simulink model "crane_model_v02_sim_improved"  (R2021a)
settings: Solver=ode23t  StartTime=0.0  StopTime=120.0  RelTol=1e-3
model workspace (MAT data in the model file):
  I_xx_0 = Simulink.Parameter
  I_xx_0.Value = 300
  I_xx_0.DataType = 'auto'
  I_xx_0.DocUnits = 'kg*m*m'
  I_xx_0.Dimensions = [1 1]
  I_xx_1 = Simulink.Parameter
  I_xx_1.Value = 336.25
  I_xx_1.DataType = 'auto'
  I_xx_1.DocUnits = 'kg*m*m'
  I_xx_1.Dimensions = [1 1]
  I_xx_2 = Simulink.Parameter
  I_xx_2.Value = 313.83
  I_xx_2.DataType = 'auto'
  I_xx_2.DocUnits = 'kg*m*m'
  I_xx_2.Dimensions = [1 1]
  I_xx_b = Simulink.Parameter
  I_xx_b.Value = 12.917
  I_xx_b.DataType = 'auto'
  I_xx_b.DocUnits = 'kg*m*m'
  I_xx_b.Dimensions = [1 1]
  I_xx_b1 = Simulink.Parameter
  I_xx_b1.Value = 10.905
  I_xx_b1.DataType = 'auto'
  I_xx_b1.Dimensions = [1 1]
  I_xx_b2 = Simulink.Parameter
  I_xx_b2.Value = 7.1406
  I_xx_b2.DataType = 'auto'
  I_xx_b2.Dimensions = [1 1]
  I_xx_c1 = Simulink.Parameter
  I_xx_c1.Value = 4.2383
  I_xx_c1.DataType = 'auto'
  I_xx_c1.Dimensions = [1 1]
  I_xx_c2 = Simulink.Parameter
  I_xx_c2.Value = 2.474
  I_xx_c2.DataType = 'auto'
  I_xx_c2.Dimensions = [1 1]
  I_yy_0 = Simulink.Parameter
  I_yy_0.Value = 300
  I_yy_0.DataType = 'auto'
  I_yy_0.DocUnits = 'kg*m*m'
  I_yy_0.Dimensions = [1 1]
  I_yy_1 = Simulink.Parameter
  I_yy_1.Value = 336.25
  I_yy_1.DataType = 'auto'
  I_yy_1.DocUnits = 'kg*m*m'
  I_yy_1.Dimensions = [1 1]
  I_yy_2 = Simulink.Parameter
  I_yy_2.Value = 313.83
  I_yy_2.DataType = 'auto'
  I_yy_2.DocUnits = 'kg*m*m'
  I_yy_2.Dimensions = [1 1]
  I_yy_b = Simulink.Parameter
  I_yy_b.Value = 12.917
  I_yy_b.DataType = 'auto'
  I_yy_b.DocUnits = 'kg*m*m'
  I_yy_b.Dimensions = [1 1]
  I_yy_b1 = Simulink.Parameter
  I_yy_b1.Value = 10.905
  I_yy_b1.DataType = 'auto'
  I_yy_b1.Dimensions = [1 1]
  I_yy_b2 = Simulink.Parameter
  I_yy_b2.Value = 7.1406
  I_yy_b2.DataType = 'auto'
  I_yy_b2.Dimensions = [1 1]
  I_yy_c1 = Simulink.Parameter
  I_yy_c1.Value = 4.2383
  I_yy_c1.DataType = 'auto'
  I_yy_c1.Dimensions = [1 1]
  I_yy_c2 = Simulink.Parameter
  I_yy_c2.Value = 2.474
  I_yy_c2.DataType = 'auto'
  I_yy_c2.Dimensions = [1 1]
  I_zz_0 = Simulink.Parameter
  I_zz_0.Value = 12
  I_zz_0.DataType = 'auto'
  I_zz_0.DocUnits = 'kg*m*m'
  I_zz_0.Dimensions = [1 1]
  I_zz_1 = Simulink.Parameter
  I_zz_1.Value = 11.25
  I_zz_1.DataType = 'auto'
  I_zz_1.DocUnits = 'kg*m*m'
  I_zz_1.Dimensions = [1 1]
  I_zz_2 = Simulink.Parameter
  I_zz_2.Value = 10.5
  I_zz_2.DataType = 'auto'
  I_zz_2.DocUnits = 'kg*m*m'
  I_zz_2.Dimensions = [1 1]
  I_zz_b = Simulink.Parameter
  I_zz_b.Value = 11.25
  I_zz_b.DataType = 'auto'
  I_zz_b.DocUnits = 'kg*m*m'
  I_zz_b.Dimensions = [1 1]
  I_zz_b1 = Simulink.Parameter
  I_zz_b1.Value = 0.16276
  I_zz_b1.DataType = 'auto'
  I_zz_b1.Dimensions = [1 1]
  I_zz_b2 = Simulink.Parameter
  I_zz_b2.Value = 0.13021
  I_zz_b2.DataType = 'auto'
  I_zz_b2.Dimensions = [1 1]
  I_zz_c1 = Simulink.Parameter
  I_zz_c1.Value = 0.16276
  I_zz_c1.DataType = 'auto'
  I_zz_c1.Dimensions = [1 1]
  I_zz_c2 = Simulink.Parameter
  I_zz_c2.Value = 0.13021
  I_zz_c2.DataType = 'auto'
  I_zz_c2.Dimensions = [1 1]
  J_a = Simulink.Parameter
  J_a.Value = 3.125
  J_a.DataType = 'auto'
  J_a.DocUnits = 'kg*m*m'
  J_a.Dimensions = [1 1]
  Sig = Simulink.Signal
  Sig.DataType = 'auto'
  Sig.Dimensions = -1
  Sig.DimensionsMode = 'auto'
  Sig.Complexity = 'auto'
  Sig.SampleTime = -1
  Sig.SamplingMode = 'auto'
  Sig1 = Simulink.Signal
  Sig1.DataType = 'auto'
  Sig1.Dimensions = -1
  Sig1.DimensionsMode = 'auto'
  Sig1.Complexity = 'auto'
  Sig1.SampleTime = -1
  Sig1.SamplingMode = 'auto'
  a1_l = Simulink.Parameter
  a1_l.Value = Simulink.data.Expression
  a1_l.Value.ExpressionString = "sqrt((l_0-h_base-l_b4y)^2+(l_b4x-l_b1x)^2)"
  a1_l.DataType = 'auto'
  a1_l.Dimensions = -1
  a1_t = Simulink.Parameter
  a1_t.Value = Simulink.data.Expression
  a1_t.Value.ExpressionString = "atan((l_0-h_base-l_b4y)/(l_b4x-l_b1x))"
  a1_t.DataType = 'auto'
  a1_t.Dimensions = -1
  a2_l = Simulink.Parameter
  a2_l.Value = Simulink.data.Expression
  a2_l.Value.ExpressionString = "sqrt((l_c1x-l_c3y)^2+(l_c3x-l_c1y)^2)"
  a2_l.DataType = 'auto'
  a2_l.Dimensions = -1
  a2_t = Simulink.Parameter
  a2_t.Value = Simulink.data.Expression
  a2_t.Value.ExpressionString = "atan((l_c1x-l_c3y)/(l_c3x-l_c1y))"
  a2_t.DataType = 'auto'
  a2_t.Dimensions = -1
  arm_d = Simulink.Parameter
  arm_d.Value = 0.3
  arm_d.DataType = 'auto'
  arm_d.DocUnits = 'm'
  arm_d.Dimensions = [1 1]
  arm_w = Simulink.Parameter
  arm_w.Value = 0.3
  arm_w.DataType = 'auto'
  arm_w.DocUnits = 'm'
  arm_w.Dimensions = [1 1]
  b_1 = Simulink.Parameter
  b_1.Value = Simulink.data.Expression
  b_1.Value.ExpressionString = "sqrt(l_b1x^2+(l_0-l_b1x)^2)"
  b_1.DataType = 'auto'
  b_1.DocUnits = 'm'
  b_1.Dimensions = -1
  b_2 = Simulink.Parameter
  b_2.Value = Simulink.data.Expression
  b_2.Value.ExpressionString = "sqrt(l_c3x^2+l_c3y^2)"
  b_2.DataType = 'auto'
  b_2.DocUnits = 'm'
  b_2.Dimensions = -1
  h_base = Simulink.Parameter
  h_base.Value = 0.2
  h_base.DataType = 'auto'
  h_base.DocUnits = 'm'
  h_base.Dimensions = [1 1]
  l_0 = Simulink.Parameter
  l_0.Value = 2.1
  l_0.DataType = 'auto'
  l_0.DocUnits = 'm'
  l_0.Dimensions = [1 1]
  l_1 = Simulink.Parameter
  l_1.Value = 2.3
  l_1.DataType = 'auto'
  l_1.DocUnits = 'm'
  l_1.Dimensions = [1 1]
  l_2 = Simulink.Parameter
  l_2.Value = 2.1
  l_2.DataType = 'auto'
  l_2.DocUnits = 'm'
  l_2.Dimensions = [1 1]
  l_a1_rod = Simulink.Parameter
  l_a1_rod.Value = Simulink.data.Expression
  l_a1_rod.Value.ExpressionString = "a1_l-l_b2"
  l_a1_rod.DataType = 'auto'
  l_a1_rod.DocUnits = 'm'
  l_a1_rod.Dimensions = -1
  l_a2_rod = Simulink.Parameter
  l_a2_rod.Value = Simulink.data.Expression
  l_a2_rod.Value.ExpressionString = "a2_l-l_c2"
  l_a2_rod.DataType = 'auto'
  l_a2_rod.DocUnits = 'm'
  l_a2_rod.Dimensions = -1
  l_b1x = Simulink.Parameter
  l_b1x.Value = 0.3
  l_b1x.DataType = 'auto'
  l_b1x.DocUnits = 'm'
  l_b1x.Dimensions = [1 1]
  l_b1z = Simulink.Parameter
  l_b1z.Value = 0.2
  l_b1z.DataType = 'auto'
  l_b1z.DocUnits = 'm'
  l_b1z.Dimensions = [1 1]
  l_b2 = Simulink.Parameter
  l_b2.Value = 1
  l_b2.DataType = 'auto'
  l_b2.DocUnits = 'm'
  l_b2.Dimensions = [1 1]
  l_b4x = Simulink.Parameter
  l_b4x.Value = 0.5
  l_b4x.DataType = 'auto'
  l_b4x.DocUnits = 'm'
  l_b4x.Dimensions = [1 1]
  l_b4y = Simulink.Parameter
  l_b4y.Value = 0.15
  l_b4y.DataType = 'auto'
  l_b4y.DocUnits = 'm'
  l_b4y.Dimensions = [1 1]
  l_c1x = Simulink.Parameter
  l_c1x.Value = 1.1
  l_c1x.DataType = 'auto'
  l_c1x.DocUnits = 'm'
  l_c1x.Dimensions = [1 1]
  l_c1y = Simulink.Parameter
  l_c1y.Value = 0.15
  l_c1y.DataType = 'auto'
  l_c1y.DocUnits = 'm'
  l_c1y.Dimensions = [1 1]
  l_c2 = Simulink.Parameter
  l_c2.Value = 0.6
  l_c2.DataType = 'auto'
  l_c2.DocUnits = 'm'
  l_c2.Dimensions = [1 1]
  l_c3x = Simulink.Parameter
  l_c3x.Value = 0.65
  l_c3x.DataType = 'auto'
  l_c3x.DocUnits = 'm'
  l_c3x.Dimensions = [1 1]
  l_c3y = Simulink.Parameter
  l_c3y.Value = 0.15
  l_c3y.DataType = 'auto'
  l_c3y.DocUnits = 'm'
  l_c3y.Dimensions = [1 1]
  l_set = 0.5
  m_0 = Simulink.Parameter
  m_0.Value = 800
  m_0.DataType = 'auto'
  m_0.DocUnits = 'kg'
  m_0.Dimensions = [1 1]
  m_1 = Simulink.Parameter
  m_1.Value = 750
  m_1.DataType = 'auto'
  m_1.DocUnits = 'kg'
  m_1.Dimensions = [1 1]
  m_2 = Simulink.Parameter
  m_2.Value = 700
  m_2.DataType = 'auto'
  m_2.DocUnits = 'kg'
  m_2.Dimensions = [1 1]
  m_b1 = Simulink.Parameter
  m_b1.Value = 125
  m_b1.DataType = 'auto'
  m_b1.DocUnits = 'kg'
  m_b1.Dimensions = [1 1]
  m_b2 = Simulink.Parameter
  m_b2.Value = 100
  m_b2.DataType = 'auto'
  m_b2.DocUnits = 'kg'
  m_b2.Dimensions = [1 1]
  m_base = Simulink.Parameter
  m_base.Value = 500
  m_base.DataType = 'auto'
  m_base.DocUnits = 'kg'
  m_base.Dimensions = [1 1]
  m_c1 = Simulink.Parameter
  m_c1.Value = 125
  m_c1.DataType = 'auto'
  m_c1.DocUnits = 'kg'
  m_c1.Dimensions = [1 1]
  m_c2 = Simulink.Parameter
  m_c2.Value = 100
  m_c2.DataType = 'auto'
  m_c2.DocUnits = 'kg'
  m_c2.Dimensions = [1 1]
  m_p = Simulink.Parameter
  m_p.Value = 2000
  m_p.DataType = 'auto'
  m_p.DocUnits = 'kg'
  m_p.Dimensions = [1 1]
  r_base = Simulink.Parameter
  r_base.Value = 0.3
  r_base.DataType = 'auto'
  r_base.DocUnits = 'm'
  r_base.Dimensions = [1 1]
  r_cyl = Simulink.Parameter
  r_cyl.Value = 0.125
  r_cyl.DataType = 'auto'
  r_cyl.DocUnits = 'm'
  r_cyl.Dimensions = [1 1]
  r_cyl_0 = Simulink.Parameter
  r_cyl_0.Value = 0.1
  r_cyl_0.DataType = 'auto'
  r_cyl_0.Dimensions = [1 1]
  x_set = 3.7
  y_set = 0.3
  z_set = 2.2
undefined symbols (not defined in the file): sigbuilder_block, X, Y, Z
libraries: sm_lib x103, nesl_utility x23, pid_lib x7, fuzblock x1
(part 1 of 5)
settings Model: OrderedModelArguments=off  Creator=jjmoey  LastModifiedBy=jjmoey

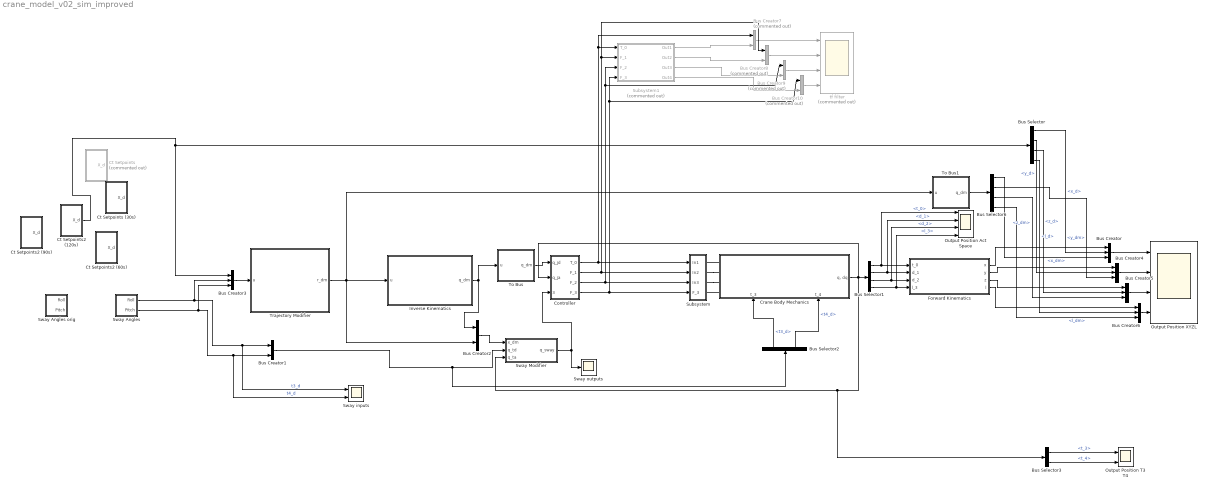
== system crane_model_v02_sim_improved ==
  Bus Creator{,3..6} (5 alike) : BusCreator  Inputs=3
  Bus Creator1 : BusCreator  Inputs=2
  Bus Creator{7..10} (4 alike) : BusCreator  Commented=on  Inputs=2
  Bus Creator2 : BusCreator  Inputs=2
  Bus Selector : BusSelector  OutputSignals=x_d,y_d,z_d,l_d
  Bus Selector1 : BusSelector  OutputSignals=t_0,d_1,d_2,l_3
  Bus Selector2 : BusSelector  OutputSignals=t3_d,t4_d
  Bus Selector3 : BusSelector  OutputSignals=t_3,t_4
  Bus Selector6 : BusSelector  OutputSignals=x_dm,y_dm,z_dm,l_dm
  Controller : Subsystem
  Crane Body Mechanics : Subsystem
      settings: PortSchema="{\"entries\":[{\"content\":{\"sides\":[{\"content\":{\"connectorIds\":[\"LConn1\",\"LConn2\",\"LConn3\",\"LConn4\"]},\"type\":\"ConnectorPlacement.EquallySpacedRectSide\",\"uuid\":\"3c12a75b-c014-4331-843e-93cd976182ad\"},{\"content\":{\"connectorIds\":[\"Out1\"],\"side\":\"RIGHT\"},\"type\":\"ConnectorPlacement.EquallySpacedRectSide\",\"uuid\":\"f6a8e3a7-cb13-4e9f-a0f7-1b13ae567996\"},{\"content\":{\"connectorIds\":[],\"side\":\"TOP\"},\"type\":\"ConnectorPlacement.EquallySpacedRectSide\",\"uuid\":\"21d4657c-d1b0-4888-a00c-4d42a03474ee\"},{\"content\":{\"connectorIds\":[\"In1\",\"In2\"],\"side\":\"BOTTOM\"},\"type\":\"ConnectorPlacement.EquallySpacedRectSide\",\"uuid\":\"dc246dea-fc9c-4a87-b817-efe1b28a592a\"}]},\"type\":\"ConnectorPlacement.EquallySpacedConnector\",\"uuid\":\"e18ee79d-7142-4697-ae33-8ae8c5e54180\"}],\"packageUris\":[\"http://schema.mathworks.com/mf0/Connector/R2020b\"],\"version\":\"1.0\"}"
  Ct Setpoints : Subsystem  Commented=on
  Ct Setpoints (30s) : Subsystem
  Ct Setpoints2 (120s) : Subsystem
  Ct Setpoints2 (60s) : Subsystem
  Ct Setpoints2 (90s) : Subsystem
  Forward Kinematics : MATLAB Function  TreatAsAtomicUnit=on
  Inverse Kinematics : MATLAB Function  TreatAsAtomicUnit=on
  Output Position Act Space : Scope  NumInputPorts=4
  Output Position T3 T4 : Scope  NumInputPorts=2
  Output Position XYZL : Scope  NumInputPorts=4
  Subsystem : Subsystem
  Subsystem1 : Subsystem  Commented=on
  Sway Angles : Subsystem
  Sway Angles orig : Subsystem
  Sway Modifier : Subsystem
  Sway inputs : Scope  NumInputPorts=2
  Sway outputs : Scope
  To Bus : Subsystem
  To Bus1 : Subsystem
  Trajectory Modifier : MATLAB Function  TreatAsAtomicUnit=on
  tf filter : Scope  Commented=on  NumInputPorts=4
  wires:
  Sway Angles/1(Roll) -> Bus Creator3/2, Sway inputs/1, Bus Creator1/1  "t3_d"
  Sway Angles/2(Pitch) -> Bus Creator3/3, Sway inputs/2, Bus Creator1/2  "t4_d"
  Ct Setpoints2 (120s)/1(X_d) -> Bus Creator3/1, Bus Selector/1
  Inverse Kinematics/1(q_dm) -> To Bus/1(u), Bus Creator2/1
  Crane Body Mechanics/1("q, dq") -> Bus Selector3/1, Sway Modifier/3(q_ta), Controller/2(q_ja), Bus Selector1/1
  Bus Selector1/1 -> Output Position Act Space/1, Forward Kinematics/1(t_0)  "<t_0>"
  Bus Selector1/2 -> Output Position Act Space/2, Forward Kinematics/2(d_1)  "<d_1>"
  Bus Selector1/3 -> Output Position Act Space/3, Forward Kinematics/3(d_2)  "<d_2>"
  Bus Selector1/4 -> Output Position Act Space/4, Forward Kinematics/4(l_3)  "<l_3>"
  Bus Creator2/1 -> Sway Modifier/1(x_dm)
  Sway Modifier/1(q_sway) -> Sway outputs/1, Controller/3(q_sway)
  Bus Creator3/1 -> Trajectory Modifier/1(u)
  To Bus/1(q_dm) -> Controller/1(q_jd)
  Trajectory Modifier/1(r_dm) -> Bus Creator2/2, To Bus1/1(u), Inverse Kinematics/1(u)
  Forward Kinematics/1(x) -> Bus Creator/1
  Bus Selector/1 -> Bus Creator/2  "<x_d>"
  Bus Selector6/1 -> Bus Creator/3  "<x_dm>"
  To Bus1/1(q_dm) -> Bus Selector6/1
  Bus Creator/1 -> Output Position XYZL/1
  Bus Creator6/1 -> Output Position XYZL/4
  Bus Creator5/1 -> Output Position XYZL/3
  Bus Creator4/1 -> Output Position XYZL/2
  Bus Selector/2 -> Bus Creator4/2  "<y_d>"
  Bus Selector6/2 -> Bus Creator4/3  "<y_dm>"
  Forward Kinematics/2(y) -> Bus Creator4/1
  Forward Kinematics/3(z) -> Bus Creator5/1
  Bus Selector6/3 -> Bus Creator5/3  "<z_dm>"
  Bus Selector/3 -> Bus Creator5/2  "<z_d>"
  Forward Kinematics/4(l) -> Bus Creator6/1
  Bus Selector/4 -> Bus Creator6/2  "<l_d>"
  Bus Selector6/4 -> Bus Creator6/3  "<l_dm>"
  Bus Creator1/1 -> Bus Selector2/1, Sway Modifier/2(q_td)
  Bus Selector2/1 -> Crane Body Mechanics/1(t_3)  "<t3_d>"
  Bus Selector2/2 -> Crane Body Mechanics/2(t_4)  "<t4_d>"
  Bus Selector3/1 -> Output Position T3 T4/1  "<t_3>"
  Bus Selector3/2 -> Output Position T3 T4/2  "<t_4>"
  Bus Creator10/1 -> tf filter/4
  Bus Creator9/1 -> tf filter/3
  Bus Creator8/1 -> tf filter/2
  Bus Creator7/1 -> tf filter/1
  Controller/1(T_0) -> Bus Creator7/1, Subsystem1/1(T_0), Subsystem/1(In1)
  Controller/2(F_1) -> Bus Creator8/1, Subsystem1/2(F_1), Subsystem/2(In2)
  Controller/3(F_2) -> Subsystem1/3(F_2), Bus Creator9/1, Subsystem/3(In3)
  Controller/4(F_3) -> Subsystem1/4(F_3), Bus Creator10/1, Subsystem/4(F_3)
  Subsystem1/1(Out1) -> Bus Creator7/2
  Subsystem1/2(Out2) -> Bus Creator8/2
  Subsystem1/3(Out3) -> Bus Creator9/2
  Subsystem1/4(Out4) -> Bus Creator10/2
  connections:
  Crane Body Mechanics/LConn1 -- Subsystem/RConn1
  Subsystem/RConn3 -- Crane Body Mechanics/LConn3
  Subsystem/RConn2 -- Crane Body Mechanics/LConn2
  Crane Body Mechanics/LConn4 -- Subsystem/RConn4

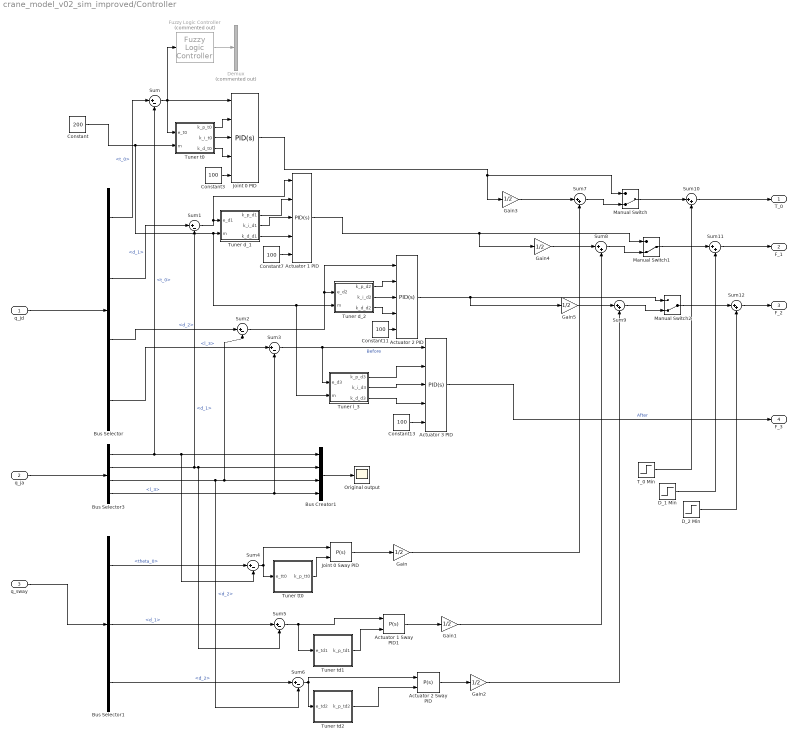
== system crane_model_v02_sim_improved/Controller ==
  q_jd : Inport
  q_ja : Inport  Port=2
  q_sway : Inport  Port=3
  Actuator 1 PID : pid_lib/PID Controller  Controller=PID  Form=Parallel  TimeDomain=Continuous-time  UseExternalTs=off  SampleTime=-1  IntegratorMethod=Forward Euler  FilterMethod=Forward Euler  ControllerParametersSource=external  P=1e6  I=1e6  D=1e6  UseFilter=on  N=100  TunerSelectOption=Transfer Function Based (PID Tuner App)  InitialConditionSource=internal  InitialConditionForIntegrator=0  InitialConditionForFilter=0  DifferentiatorICPrevScaledInput=0  ExternalReset=none  TrackingMode=off  Kt=1  LimitOutput=off  SatLimitsSource=internal  UpperSaturationLimit=inf  LowerSaturationLimit=-inf  LinearizeAsGain=on  AntiWindupMode=none  Kb=1  POutMin=[]  POutMax=[]  IOutMin=[]  IOutMax=[]  DOutMin=[]  DOutMax=[]  NOutMin=[]  NOutMax=[]  SumOutMin=[]  SumOutMax=[]  SaturationOutMin=[]  SaturationOutMax=[]  PParamMin=[]  PParamMax=[]  IParamMin=[]  IParamMax=[]  DParamMin=[]  DParamMax=[]  NParamMin=[]  NParamMax=[]  KbParamMin=[]  KbParamMax=[]  KtParamMin=[]  KtParamMax=[]  KbOutMin=[]  KbOutMax=[]  KtOutMin=[]  KtOutMax=[]  IntegratorOutMin=[]  IntegratorOutMax=[]  FilterOutMin=[]  FilterOutMax=[]  SumI1OutMin=[]  SumI1OutMax=[]  SumI2OutMin=[]  SumI2OutMax=[]  SumI3OutMin=[]  SumI3OutMax=[]  SumI4OutMin=[]  SumI4OutMax=[]  SumDOutMin=[]  SumDOutMax=[]  DifferentiatorOutMin=[]  DifferentiatorOutMax=[]  FilterDiffOutCoefMin=[]  FilterDiffOutCoefMax=[]  ReciprocalOutMin=[]  ReciprocalOutMax=[]  SumDenOutMin=[]  SumDenOutMax=[]  SumNumOutMin=[]  SumNumOutMax=[]  DivideOutMin=[]  DivideOutMax=[]  UdiffTsProdOutMin=[]  UdiffTsProdOutMax=[]  NTsProdOutMin=[]  NTsProdOutMax=[]  UintegralTsProdOutMin=[]  UintegralTsProdOutMax=[]  UngainTsProdOutMin=[]  UngainTsProdOutMax=[]  IntegratorContinuousStateAttributes=''  IntegratorStateMustResolveToSignalObject=off  IntegratorRTWStateStorageClass=Auto  FilterContinuousStateAttributes=''  FilterStateMustResolveToSignalObject=off  FilterRTWStateStorageClass=Auto  ParallelPVariant=ExternalParameters  IdealPVariant=Disabled  IVariant=ExternalParameters  DVariant=ExternalParameters  IntegratorVariant=Continuous  SatVariant=Disabled  AWVariant=Passthrough  PCopyVariant=Disabled  TRVariant=Disabled  FdbkBlocksVariant=Forward  IdealPFdbkVariant=Disabled  SatFdbkVariant=Disabled  DerivativeFilterVariant=ContFilter  NVariant=ExternalParameters  NCopyVariant=Disabled  FilterICVariant=InternalICsFilter  IntegratorICVariant=InternalICs  ExternalResetVariant=Disabled  TRSumVariant=Passthrough  SumFdbkVariant=Disabled  SumVariant=Sum_PID  TsampFilterVariant=InternalTs  TsampNgainVariant=Passthrough  TsampIntegralVariant=Passthrough  ExternalSaturationOutDataTypeStr=Inherit: Same as second input
  Actuator 1 Sway PID1 : pid_lib/PID Controller  Controller=P  Form=Parallel  TimeDomain=Continuous-time  UseExternalTs=off  SampleTime=-1  IntegratorMethod=Forward Euler  FilterMethod=Forward Euler  ControllerParametersSource=external  P=2.5e5  I=5e4  D=5e5  UseFilter=on  N=100  TunerSelectOption=Transfer Function Based (PID Tuner App)  InitialConditionSource=internal  InitialConditionForIntegrator=0  InitialConditionForFilter=0  DifferentiatorICPrevScaledInput=0  ExternalReset=none  TrackingMode=off  Kt=1  LimitOutput=off  SatLimitsSource=internal  UpperSaturationLimit=inf  LowerSaturationLimit=-inf  LinearizeAsGain=on  AntiWindupMode=none  Kb=1  POutMin=[]  POutMax=[]  IOutMin=[]  IOutMax=[]  DOutMin=[]  DOutMax=[]  NOutMin=[]  NOutMax=[]  SumOutMin=[]  SumOutMax=[]  SaturationOutMin=[]  SaturationOutMax=[]  PParamMin=[]  PParamMax=[]  IParamMin=[]  IParamMax=[]  DParamMin=[]  DParamMax=[]  NParamMin=[]  NParamMax=[]  KbParamMin=[]  KbParamMax=[]  KtParamMin=[]  KtParamMax=[]  KbOutMin=[]  KbOutMax=[]  KtOutMin=[]  KtOutMax=[]  IntegratorOutMin=[]  IntegratorOutMax=[]  FilterOutMin=[]  FilterOutMax=[]  SumI1OutMin=[]  SumI1OutMax=[]  SumI2OutMin=[]  SumI2OutMax=[]  SumI3OutMin=[]  SumI3OutMax=[]  SumI4OutMin=[]  SumI4OutMax=[]  SumDOutMin=[]  SumDOutMax=[]  DifferentiatorOutMin=[]  DifferentiatorOutMax=[]  FilterDiffOutCoefMin=[]  FilterDiffOutCoefMax=[]  ReciprocalOutMin=[]  ReciprocalOutMax=[]  SumDenOutMin=[]  SumDenOutMax=[]  SumNumOutMin=[]  SumNumOutMax=[]  DivideOutMin=[]  DivideOutMax=[]  UdiffTsProdOutMin=[]  UdiffTsProdOutMax=[]  NTsProdOutMin=[]  NTsProdOutMax=[]  UintegralTsProdOutMin=[]  UintegralTsProdOutMax=[]  UngainTsProdOutMin=[]  UngainTsProdOutMax=[]  IntegratorContinuousStateAttributes=''  IntegratorStateMustResolveToSignalObject=off  IntegratorRTWStateStorageClass=Auto  FilterContinuousStateAttributes=''  FilterStateMustResolveToSignalObject=off  FilterRTWStateStorageClass=Auto  ParallelPVariant=ExternalParameters  IdealPVariant=Disabled  IVariant=Disabled  DVariant=Disabled  IntegratorVariant=Disabled  SatVariant=Disabled  AWVariant=Disabled  PCopyVariant=Disabled  TRVariant=Disabled  FdbkBlocksVariant=Forward  IdealPFdbkVariant=Disabled  SatFdbkVariant=Disabled  DerivativeFilterVariant=Disabled  NVariant=Disabled  NCopyVariant=Disabled_SignalSpec  FilterICVariant=Disabled  IntegratorICVariant=Disabled  ExternalResetVariant=Disabled  TRSumVariant=Passthrough  SumFdbkVariant=Disabled  SumVariant=Passthrough_P  TsampFilterVariant=InternalTs  TsampNgainVariant=Passthrough  TsampIntegralVariant=Disabled_SignalSpec  ExternalSaturationOutDataTypeStr=Inherit: Same as second input
  Actuator 2 PID : pid_lib/PID Controller  Controller=PID  Form=Parallel  TimeDomain=Continuous-time  UseExternalTs=off  SampleTime=-1  IntegratorMethod=Forward Euler  FilterMethod=Forward Euler  ControllerParametersSource=external  P=7.5e4  I=2.5e4  D=7.5e4  UseFilter=on  N=100  TunerSelectOption=Transfer Function Based (PID Tuner App)  InitialConditionSource=internal  InitialConditionForIntegrator=0  InitialConditionForFilter=0  DifferentiatorICPrevScaledInput=0  ExternalReset=none  TrackingMode=off  Kt=1  LimitOutput=off  SatLimitsSource=internal  UpperSaturationLimit=inf  LowerSaturationLimit=-inf  LinearizeAsGain=on  AntiWindupMode=none  Kb=1  POutMin=[]  POutMax=[]  IOutMin=[]  IOutMax=[]  DOutMin=[]  DOutMax=[]  NOutMin=[]  NOutMax=[]  SumOutMin=[]  SumOutMax=[]  SaturationOutMin=[]  SaturationOutMax=[]  PParamMin=[]  PParamMax=[]  IParamMin=[]  IParamMax=[]  DParamMin=[]  DParamMax=[]  NParamMin=[]  NParamMax=[]  KbParamMin=[]  KbParamMax=[]  KtParamMin=[]  KtParamMax=[]  KbOutMin=[]  KbOutMax=[]  KtOutMin=[]  KtOutMax=[]  IntegratorOutMin=[]  IntegratorOutMax=[]  FilterOutMin=[]  FilterOutMax=[]  SumI1OutMin=[]  SumI1OutMax=[]  SumI2OutMin=[]  SumI2OutMax=[]  SumI3OutMin=[]  SumI3OutMax=[]  SumI4OutMin=[]  SumI4OutMax=[]  SumDOutMin=[]  SumDOutMax=[]  DifferentiatorOutMin=[]  DifferentiatorOutMax=[]  FilterDiffOutCoefMin=[]  FilterDiffOutCoefMax=[]  ReciprocalOutMin=[]  ReciprocalOutMax=[]  SumDenOutMin=[]  SumDenOutMax=[]  SumNumOutMin=[]  SumNumOutMax=[]  DivideOutMin=[]  DivideOutMax=[]  UdiffTsProdOutMin=[]  UdiffTsProdOutMax=[]  NTsProdOutMin=[]  NTsProdOutMax=[]  UintegralTsProdOutMin=[]  UintegralTsProdOutMax=[]  UngainTsProdOutMin=[]  UngainTsProdOutMax=[]  IntegratorContinuousStateAttributes=''  IntegratorStateMustResolveToSignalObject=off  IntegratorRTWStateStorageClass=Auto  FilterContinuousStateAttributes=''  FilterStateMustResolveToSignalObject=off  FilterRTWStateStorageClass=Auto  ParallelPVariant=ExternalParameters  IdealPVariant=Disabled  IVariant=ExternalParameters  DVariant=ExternalParameters  IntegratorVariant=Continuous  SatVariant=Disabled  AWVariant=Passthrough  PCopyVariant=Disabled  TRVariant=Disabled  FdbkBlocksVariant=Forward  IdealPFdbkVariant=Disabled  SatFdbkVariant=Disabled  DerivativeFilterVariant=ContFilter  NVariant=ExternalParameters  NCopyVariant=Disabled  FilterICVariant=InternalICsFilter  IntegratorICVariant=InternalICs  ExternalResetVariant=Disabled  TRSumVariant=Passthrough  SumFdbkVariant=Disabled  SumVariant=Sum_PID  TsampFilterVariant=InternalTs  TsampNgainVariant=Passthrough  TsampIntegralVariant=Passthrough  ExternalSaturationOutDataTypeStr=Inherit: Same as second input
  Actuator 2 Sway PID : pid_lib/PID Controller  Controller=P  Form=Parallel  TimeDomain=Continuous-time  UseExternalTs=off  SampleTime=-1  IntegratorMethod=Forward Euler  FilterMethod=Forward Euler  ControllerParametersSource=external  P=5e4  I=5e4  D=5e5  UseFilter=on  N=100  TunerSelectOption=Transfer Function Based (PID Tuner App)  InitialConditionSource=internal  InitialConditionForIntegrator=0  InitialConditionForFilter=0  DifferentiatorICPrevScaledInput=0  ExternalReset=none  TrackingMode=off  Kt=1  LimitOutput=off  SatLimitsSource=internal  UpperSaturationLimit=inf  LowerSaturationLimit=-inf  LinearizeAsGain=on  AntiWindupMode=none  Kb=1  POutMin=[]  POutMax=[]  IOutMin=[]  IOutMax=[]  DOutMin=[]  DOutMax=[]  NOutMin=[]  NOutMax=[]  SumOutMin=[]  SumOutMax=[]  SaturationOutMin=[]  SaturationOutMax=[]  PParamMin=[]  PParamMax=[]  IParamMin=[]  IParamMax=[]  DParamMin=[]  DParamMax=[]  NParamMin=[]  NParamMax=[]  KbParamMin=[]  KbParamMax=[]  KtParamMin=[]  KtParamMax=[]  KbOutMin=[]  KbOutMax=[]  KtOutMin=[]  KtOutMax=[]  IntegratorOutMin=[]  IntegratorOutMax=[]  FilterOutMin=[]  FilterOutMax=[]  SumI1OutMin=[]  SumI1OutMax=[]  SumI2OutMin=[]  SumI2OutMax=[]  SumI3OutMin=[]  SumI3OutMax=[]  SumI4OutMin=[]  SumI4OutMax=[]  SumDOutMin=[]  SumDOutMax=[]  DifferentiatorOutMin=[]  DifferentiatorOutMax=[]  FilterDiffOutCoefMin=[]  FilterDiffOutCoefMax=[]  ReciprocalOutMin=[]  ReciprocalOutMax=[]  SumDenOutMin=[]  SumDenOutMax=[]  SumNumOutMin=[]  SumNumOutMax=[]  DivideOutMin=[]  DivideOutMax=[]  UdiffTsProdOutMin=[]  UdiffTsProdOutMax=[]  NTsProdOutMin=[]  NTsProdOutMax=[]  UintegralTsProdOutMin=[]  UintegralTsProdOutMax=[]  UngainTsProdOutMin=[]  UngainTsProdOutMax=[]  IntegratorContinuousStateAttributes=''  IntegratorStateMustResolveToSignalObject=off  IntegratorRTWStateStorageClass=Auto  FilterContinuousStateAttributes=''  FilterStateMustResolveToSignalObject=off  FilterRTWStateStorageClass=Auto  ParallelPVariant=ExternalParameters  IdealPVariant=Disabled  IVariant=Disabled  DVariant=Disabled  IntegratorVariant=Disabled  SatVariant=Disabled  AWVariant=Disabled  PCopyVariant=Disabled  TRVariant=Disabled  FdbkBlocksVariant=Forward  IdealPFdbkVariant=Disabled  SatFdbkVariant=Disabled  DerivativeFilterVariant=Disabled  NVariant=Disabled  NCopyVariant=Disabled_SignalSpec  FilterICVariant=Disabled  IntegratorICVariant=Disabled  ExternalResetVariant=Disabled  TRSumVariant=Passthrough  SumFdbkVariant=Disabled  SumVariant=Passthrough_P  TsampFilterVariant=InternalTs  TsampNgainVariant=Passthrough  TsampIntegralVariant=Disabled_SignalSpec  ExternalSaturationOutDataTypeStr=Inherit: Same as second input
  Actuator 3 PID : pid_lib/PID Controller  Controller=PID  Form=Parallel  TimeDomain=Continuous-time  UseExternalTs=off  SampleTime=-1  IntegratorMethod=Forward Euler  FilterMethod=Forward Euler  ControllerParametersSource=external  P=1.5e4  I=1.5e4  D=6.5e3  UseFilter=on  N=100  TunerSelectOption=Transfer Function Based (PID Tuner App)  InitialConditionSource=internal  InitialConditionForIntegrator=0  InitialConditionForFilter=0  DifferentiatorICPrevScaledInput=0  ExternalReset=none  TrackingMode=off  Kt=1  LimitOutput=off  SatLimitsSource=internal  UpperSaturationLimit=inf  LowerSaturationLimit=-inf  LinearizeAsGain=on  AntiWindupMode=none  Kb=1  POutMin=[]  POutMax=[]  IOutMin=[]  IOutMax=[]  DOutMin=[]  DOutMax=[]  NOutMin=[]  NOutMax=[]  SumOutMin=[]  SumOutMax=[]  SaturationOutMin=[]  SaturationOutMax=[]  PParamMin=[]  PParamMax=[]  IParamMin=[]  IParamMax=[]  DParamMin=[]  DParamMax=[]  NParamMin=[]  NParamMax=[]  KbParamMin=[]  KbParamMax=[]  KtParamMin=[]  KtParamMax=[]  KbOutMin=[]  KbOutMax=[]  KtOutMin=[]  KtOutMax=[]  IntegratorOutMin=[]  IntegratorOutMax=[]  FilterOutMin=[]  FilterOutMax=[]  SumI1OutMin=[]  SumI1OutMax=[]  SumI2OutMin=[]  SumI2OutMax=[]  SumI3OutMin=[]  SumI3OutMax=[]  SumI4OutMin=[]  SumI4OutMax=[]  SumDOutMin=[]  SumDOutMax=[]  DifferentiatorOutMin=[]  DifferentiatorOutMax=[]  FilterDiffOutCoefMin=[]  FilterDiffOutCoefMax=[]  ReciprocalOutMin=[]  ReciprocalOutMax=[]  SumDenOutMin=[]  SumDenOutMax=[]  SumNumOutMin=[]  SumNumOutMax=[]  DivideOutMin=[]  DivideOutMax=[]  UdiffTsProdOutMin=[]  UdiffTsProdOutMax=[]  NTsProdOutMin=[]  NTsProdOutMax=[]  UintegralTsProdOutMin=[]  UintegralTsProdOutMax=[]  UngainTsProdOutMin=[]  UngainTsProdOutMax=[]  IntegratorContinuousStateAttributes=''  IntegratorStateMustResolveToSignalObject=off  IntegratorRTWStateStorageClass=Auto  FilterContinuousStateAttributes=''  FilterStateMustResolveToSignalObject=off  FilterRTWStateStorageClass=Auto  ParallelPVariant=ExternalParameters  IdealPVariant=Disabled  IVariant=ExternalParameters  DVariant=ExternalParameters  IntegratorVariant=Continuous  SatVariant=Disabled  AWVariant=Passthrough  PCopyVariant=Disabled  TRVariant=Disabled  FdbkBlocksVariant=Forward  IdealPFdbkVariant=Disabled  SatFdbkVariant=Disabled  DerivativeFilterVariant=ContFilter  NVariant=ExternalParameters  NCopyVariant=Disabled  FilterICVariant=InternalICsFilter  IntegratorICVariant=InternalICs  ExternalResetVariant=Disabled  TRSumVariant=Passthrough  SumFdbkVariant=Disabled  SumVariant=Sum_PID  TsampFilterVariant=InternalTs  TsampNgainVariant=Passthrough  TsampIntegralVariant=Passthrough  ExternalSaturationOutDataTypeStr=Inherit: Same as second input
  Bus Creator1 : BusCreator  Inputs=4
  Bus Selector : BusSelector  OutputSignals=t_0,d_1,d_2,l_3
  Bus Selector1 : BusSelector  OutputSignals=theta_0,d_1,d_2
  Bus Selector3 : BusSelector  OutputSignals=t_0,d_1,d_2,l_3
  Constant : Constant  Value=200  SampleTime=[0,0]
  Constant{3,7,11,13} (4 alike) : Constant  Value=100  SampleTime=[0,0]
  D_1 Min : Step  Before=6.25e4  After=6.25e4  SampleTime=[0,0]
  D_2 Min : Step  Before=-2.5e3  After=-2.5e3  SampleTime=[0,0]
  Demux : Demux  Commented=on  Outputs=3
  Fuzzy Logic Controller : fuzblock/Fuzzy Logic  Controller  Commented=on  FIS=ctrl_t0  OutputSampleNumber=101  DataType=double  FuzzifiedInputs=off  RuleFiringStrengths=off  RuleOutputs=off  AggregatedOutputs=off  SimulateUsing=Interpreted execution  OutOfRangeInputValueMessage=warning  NoRuleFiredMessage=warning  EmptyOutputFuzzySetMessage=warning
  Gain{,1..5} (6 alike) : Gain  Gain=1/2
  Joint 0 PID : pid_lib/PID Controller  Controller=PID  Form=Parallel  TimeDomain=Continuous-time  UseExternalTs=off  SampleTime=-1  IntegratorMethod=Forward Euler  FilterMethod=Forward Euler  ControllerParametersSource=external  P=5e5  I=5e4  D=5e5  UseFilter=on  N=100  TunerSelectOption=Transfer Function Based (PID Tuner App)  InitialConditionSource=internal  InitialConditionForIntegrator=0  InitialConditionForFilter=0  DifferentiatorICPrevScaledInput=0  ExternalReset=none  TrackingMode=off  Kt=1  LimitOutput=off  SatLimitsSource=internal  UpperSaturationLimit=inf  LowerSaturationLimit=-inf  LinearizeAsGain=on  AntiWindupMode=none  Kb=1  POutMin=[]  POutMax=[]  IOutMin=[]  IOutMax=[]  DOutMin=[]  DOutMax=[]  NOutMin=[]  NOutMax=[]  SumOutMin=[]  SumOutMax=[]  SaturationOutMin=[]  SaturationOutMax=[]  PParamMin=[]  PParamMax=[]  IParamMin=[]  IParamMax=[]  DParamMin=[]  DParamMax=[]  NParamMin=[]  NParamMax=[]  KbParamMin=[]  KbParamMax=[]  KtParamMin=[]  KtParamMax=[]  KbOutMin=[]  KbOutMax=[]  KtOutMin=[]  KtOutMax=[]  IntegratorOutMin=[]  IntegratorOutMax=[]  FilterOutMin=[]  FilterOutMax=[]  SumI1OutMin=[]  SumI1OutMax=[]  SumI2OutMin=[]  SumI2OutMax=[]  SumI3OutMin=[]  SumI3OutMax=[]  SumI4OutMin=[]  SumI4OutMax=[]  SumDOutMin=[]  SumDOutMax=[]  DifferentiatorOutMin=[]  DifferentiatorOutMax=[]  FilterDiffOutCoefMin=[]  FilterDiffOutCoefMax=[]  ReciprocalOutMin=[]  ReciprocalOutMax=[]  SumDenOutMin=[]  SumDenOutMax=[]  SumNumOutMin=[]  SumNumOutMax=[]  DivideOutMin=[]  DivideOutMax=[]  UdiffTsProdOutMin=[]  UdiffTsProdOutMax=[]  NTsProdOutMin=[]  NTsProdOutMax=[]  UintegralTsProdOutMin=[]  UintegralTsProdOutMax=[]  UngainTsProdOutMin=[]  UngainTsProdOutMax=[]  IntegratorContinuousStateAttributes=''  IntegratorStateMustResolveToSignalObject=off  IntegratorRTWStateStorageClass=Auto  FilterContinuousStateAttributes=''  FilterStateMustResolveToSignalObject=off  FilterRTWStateStorageClass=Auto  ParallelPVariant=ExternalParameters  IdealPVariant=Disabled  IVariant=ExternalParameters  DVariant=ExternalParameters  IntegratorVariant=Continuous  SatVariant=Disabled  AWVariant=Passthrough  PCopyVariant=Disabled  TRVariant=Disabled  FdbkBlocksVariant=Forward  IdealPFdbkVariant=Disabled  SatFdbkVariant=Disabled  DerivativeFilterVariant=ContFilter  NVariant=ExternalParameters  NCopyVariant=Disabled  FilterICVariant=InternalICsFilter  IntegratorICVariant=InternalICs  ExternalResetVariant=Disabled  TRSumVariant=Passthrough  SumFdbkVariant=Disabled  SumVariant=Sum_PID  TsampFilterVariant=InternalTs  TsampNgainVariant=Passthrough  TsampIntegralVariant=Passthrough  ExternalSaturationOutDataTypeStr=Inherit: Same as second input
  Joint 0 Sway PID : pid_lib/PID Controller  Controller=P  Form=Parallel  TimeDomain=Continuous-time  UseExternalTs=off  SampleTime=-1  IntegratorMethod=Forward Euler  FilterMethod=Forward Euler  ControllerParametersSource=external  P=5e4  I=5e4  D=5e5  UseFilter=on  N=100  TunerSelectOption=Transfer Function Based (PID Tuner App)  InitialConditionSource=internal  InitialConditionForIntegrator=0  InitialConditionForFilter=0  DifferentiatorICPrevScaledInput=0  ExternalReset=none  TrackingMode=off  Kt=1  LimitOutput=off  SatLimitsSource=internal  UpperSaturationLimit=inf  LowerSaturationLimit=-inf  LinearizeAsGain=on  AntiWindupMode=none  Kb=1  POutMin=[]  POutMax=[]  IOutMin=[]  IOutMax=[]  DOutMin=[]  DOutMax=[]  NOutMin=[]  NOutMax=[]  SumOutMin=[]  SumOutMax=[]  SaturationOutMin=[]  SaturationOutMax=[]  PParamMin=[]  PParamMax=[]  IParamMin=[]  IParamMax=[]  DParamMin=[]  DParamMax=[]  NParamMin=[]  NParamMax=[]  KbParamMin=[]  KbParamMax=[]  KtParamMin=[]  KtParamMax=[]  KbOutMin=[]  KbOutMax=[]  KtOutMin=[]  KtOutMax=[]  IntegratorOutMin=[]  IntegratorOutMax=[]  FilterOutMin=[]  FilterOutMax=[]  SumI1OutMin=[]  SumI1OutMax=[]  SumI2OutMin=[]  SumI2OutMax=[]  SumI3OutMin=[]  SumI3OutMax=[]  SumI4OutMin=[]  SumI4OutMax=[]  SumDOutMin=[]  SumDOutMax=[]  DifferentiatorOutMin=[]  DifferentiatorOutMax=[]  FilterDiffOutCoefMin=[]  FilterDiffOutCoefMax=[]  ReciprocalOutMin=[]  ReciprocalOutMax=[]  SumDenOutMin=[]  SumDenOutMax=[]  SumNumOutMin=[]  SumNumOutMax=[]  DivideOutMin=[]  DivideOutMax=[]  UdiffTsProdOutMin=[]  UdiffTsProdOutMax=[]  NTsProdOutMin=[]  NTsProdOutMax=[]  UintegralTsProdOutMin=[]  UintegralTsProdOutMax=[]  UngainTsProdOutMin=[]  UngainTsProdOutMax=[]  IntegratorContinuousStateAttributes=''  IntegratorStateMustResolveToSignalObject=off  IntegratorRTWStateStorageClass=Auto  FilterContinuousStateAttributes=''  FilterStateMustResolveToSignalObject=off  FilterRTWStateStorageClass=Auto  ParallelPVariant=ExternalParameters  IdealPVariant=Disabled  IVariant=Disabled  DVariant=Disabled  IntegratorVariant=Disabled  SatVariant=Disabled  AWVariant=Disabled  PCopyVariant=Disabled  TRVariant=Disabled  FdbkBlocksVariant=Forward  IdealPFdbkVariant=Disabled  SatFdbkVariant=Disabled  DerivativeFilterVariant=Disabled  NVariant=Disabled  NCopyVariant=Disabled_SignalSpec  FilterICVariant=Disabled  IntegratorICVariant=Disabled  ExternalResetVariant=Disabled  TRSumVariant=Passthrough  SumFdbkVariant=Disabled  SumVariant=Passthrough_P  TsampFilterVariant=InternalTs  TsampNgainVariant=Passthrough  TsampIntegralVariant=Disabled_SignalSpec  ExternalSaturationOutDataTypeStr=Inherit: Same as second input
  Manual Switch : ManualSwitch  CurrentSetting=0
  Manual Switch1 : ManualSwitch  CurrentSetting=0
  Manual Switch2 : ManualSwitch  CurrentSetting=0
  Original output : Scope
  Sum{,1..6} (7 alike) : Sum  Inputs=|+-
  Sum{7..12} (6 alike) : Sum  Inputs=|++
  T_0 Min : Step  Before=-4.25e4  After=-4.25e4  SampleTime=[0,0]
  Tuner d_1 : MATLAB Function  TreatAsAtomicUnit=on
  Tuner d_2 : MATLAB Function  TreatAsAtomicUnit=on
  Tuner l_3 : MATLAB Function  TreatAsAtomicUnit=on
  Tuner t0 : MATLAB Function  TreatAsAtomicUnit=on
  Tuner td1 : MATLAB Function  TreatAsAtomicUnit=on
  Tuner td2 : MATLAB Function  TreatAsAtomicUnit=on
  Tuner tt0 : MATLAB Function  TreatAsAtomicUnit=on
  T_0 : Outport
  F_1 : Outport  Port=2
  F_2 : Outport  Port=3
  F_3 : Outport  Port=4
  wires:
  q_jd/1 -> Bus Selector/1
  Bus Selector/1 -> Sum/1  "<t_0>"
  Joint 0 PID/1 -> Gain3/1, Manual Switch/1
  Actuator 1 PID/1 -> Gain4/1, Manual Switch1/1
  Actuator 2 PID/1 -> Gain5/1, Manual Switch2/1
  Bus Selector/2 -> Sum1/1  "<d_1>"
  q_ja/1 -> Bus Selector3/1
  Bus Selector3/1 -> Bus Creator1/1, Sum4/2, Sum/2  "<t_0>"
  Bus Selector3/2 -> Bus Creator1/2, Sum5/2, Sum1/2  "<d_1>"
  Sum/1 -> Joint 0 PID/1, Tuner t0/1(e_t0), Fuzzy Logic Controller/1
  Sum1/1 -> Actuator 1 PID/1, Tuner d_1/1(e_d1)
  Bus Selector/3 -> Sum2/1  "<d_2>"
  Sum2/1 -> Actuator 2 PID/1, Tuner d_2/1(e_d2)
  Bus Selector3/3 -> Bus Creator1/3, Sum2/2, Sum6/2  "<d_2>"
  Bus Selector/4 -> Sum3/1  "<l_3>"
  Sum3/1 -> Tuner l_3/1(e_d3), Actuator 3 PID/1  "Before"
  Bus Selector3/4 -> Bus Creator1/4, Sum3/2  "<l_3>"
  q_sway/1 -> Bus Selector1/1
  Bus Selector1/1 -> Sum4/1  "<theta_0>"
  Bus Selector1/2 -> Sum5/1  "<d_1>"
  Bus Selector1/3 -> Sum6/1  "<d_2>"
  Sum4/1 -> Tuner tt0/1(e_tt0), Joint 0 Sway PID/1
  Sum5/1 -> Tuner td1/1(e_td1), Actuator 1 Sway PID1/1
  Sum6/1 -> Tuner td2/1(e_td2), Actuator 2 Sway PID/1
  Joint 0 Sway PID/1 -> Gain/1
  Actuator 1 Sway PID1/1 -> Gain1/1
  Actuator 2 Sway PID/1 -> Gain2/1
  Gain3/1 -> Sum7/1
  Gain4/1 -> Sum8/1
  Sum7/1 -> Manual Switch/2
  Sum8/1 -> Manual Switch1/2
  Sum9/1 -> Manual Switch2/2
  Gain/1 -> Sum7/2
  Gain1/1 -> Sum8/2
  Gain2/1 -> Sum9/2
  Manual Switch/1 -> Sum10/1
  Gain5/1 -> Sum9/1
  Manual Switch1/1 -> Sum11/1
  Manual Switch2/1 -> Sum12/1
  Actuator 3 PID/1 -> F_3/1  "After"
  Bus Creator1/1 -> Original output/1
  Constant3/1 -> Joint 0 PID/5
  Constant7/1 -> Actuator 1 PID/5
  Constant11/1 -> Actuator 2 PID/5
  Constant13/1 -> Actuator 3 PID/5
  Fuzzy Logic Controller/1 -> Demux/1
  Tuner d_1/1(k_p_d1) -> Actuator 1 PID/2
  Tuner d_1/2(k_i_d1) -> Actuator 1 PID/3
  Tuner d_1/3(k_d_d1) -> Actuator 1 PID/4
  Tuner d_2/1(k_p_d2) -> Actuator 2 PID/2
  Tuner d_2/2(k_i_d2) -> Actuator 2 PID/3
  Tuner d_2/3(k_d_d2) -> Actuator 2 PID/4
  Tuner l_3/1(k_p_d3) -> Actuator 3 PID/2
  Tuner l_3/2(k_i_d3) -> Actuator 3 PID/3
  Tuner l_3/3(k_d_d3) -> Actuator 3 PID/4
  Tuner t0/1(k_p_t0) -> Joint 0 PID/2
  Tuner t0/2(k_i_t0) -> Joint 0 PID/3
  Tuner t0/3(k_d_t0) -> Joint 0 PID/4
  Tuner tt0/1(k_p_tt0) -> Joint 0 Sway PID/2
  Tuner td1/1(k_p_td1) -> Actuator 1 Sway PID1/2
  Tuner td2/1(k_p_td2) -> Actuator 2 Sway PID/2
  Sum10/1 -> T_0/1
  T_0 Min/1 -> Sum10/2
  Sum11/1 -> F_1/1
  Sum12/1 -> F_2/1
  D_1 Min/1 -> Sum11/2
  D_2 Min/1 -> Sum12/2
  Constant/1 -> Tuner l_3/2(m), Tuner d_2/2(m), Tuner d_1/2(m), Tuner t0/2(m)
